simulink model "Kinematics"  (R2022b)
settings: Solver=VariableStepAuto  StartTime=0.0  StopTime=10.0  RelTol=1e-3
libraries: simulink_extras x4
settings Model: Creator=Kumar  LastModifiedBy=Kumar

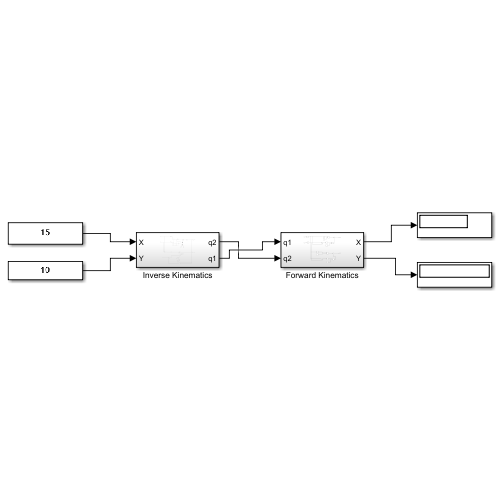
[thumbnail: Simulink's stored preview of the top-level diagram]
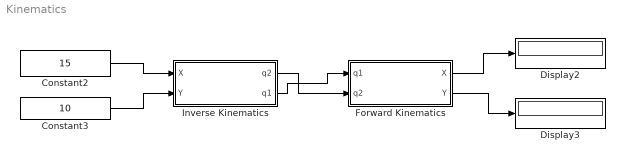
== system Kinematics ==
  Constant2 : Constant  Value=15
  Constant3 : Constant  Value=10
  Display2 : Display
      settings: Format=decimal (Stored Integer)  Decimation=2
  Display3 : Display
      settings: Decimation=2
  Forward Kinematics : Subsystem
  Inverse Kinematics : Subsystem
  wires:
  Constant3/1 -> Inverse Kinematics/2(Y)
  Constant2/1 -> Inverse Kinematics/1(X)
  Forward Kinematics/1(X) -> Display2/1
  Forward Kinematics/2(Y) -> Display3/1
  Inverse Kinematics/1(q2) -> Forward Kinematics/2(q2)
  Inverse Kinematics/2(q1) -> Forward Kinematics/1(q1)

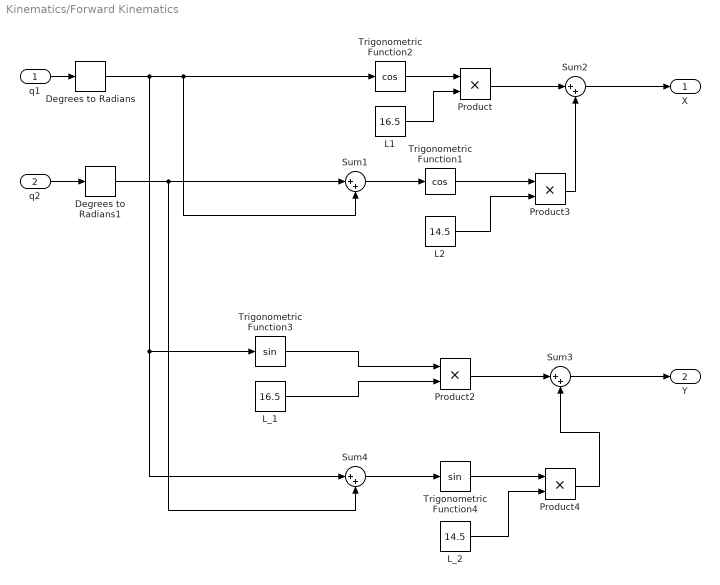
== system Kinematics/Forward Kinematics ==
  q1 : Inport
  q2 : Inport  Port=2
  Degrees to Radians : simulink_extras/Transformations/Degrees to Radians
  Degrees to Radians1 : simulink_extras/Transformations/Degrees to Radians
  L1 : Constant  Value=16.5
  L2 : Constant  Value=14.5
  L_1 : Constant  Value=16.5
  L_2 : Constant  Value=14.5
  Product{,2..4} (4 alike) : Product
  Sum{1..4} (4 alike) : Sum  Inputs=|++
  Trigonometric Function1 : Trigonometry  Operator=cos
  Trigonometric Function2 : Trigonometry  Operator=cos
  Trigonometric Function3 : Trigonometry
  Trigonometric Function4 : Trigonometry
  X : Outport
  Y : Outport  Port=2
  wires:
  Trigonometric Function3/1 -> Product2/1
  q1/1 -> Degrees to Radians/1
  q2/1 -> Degrees to Radians1/1
  Trigonometric Function2/1 -> Product/1
  Trigonometric Function1/1 -> Product3/1
  L1/1 -> Product/2
  Product/1 -> Sum2/1
  L2/1 -> Product3/2
  Product3/1 -> Sum2/2
  Sum1/1 -> Trigonometric Function1/1
  Product2/1 -> Sum3/1
  L_1/1 -> Product2/2
  Sum4/1 -> Trigonometric Function4/1
  Trigonometric Function4/1 -> Product4/1
  Product4/1 -> Sum3/2
  L_2/1 -> Product4/2
  Degrees to Radians/1 -> Trigonometric Function2/1, Sum1/2, Sum4/1, Trigonometric Function3/1
  Degrees to Radians1/1 -> Sum4/2, Sum1/1
  Sum2/1 -> X/1
  Sum3/1 -> Y/1

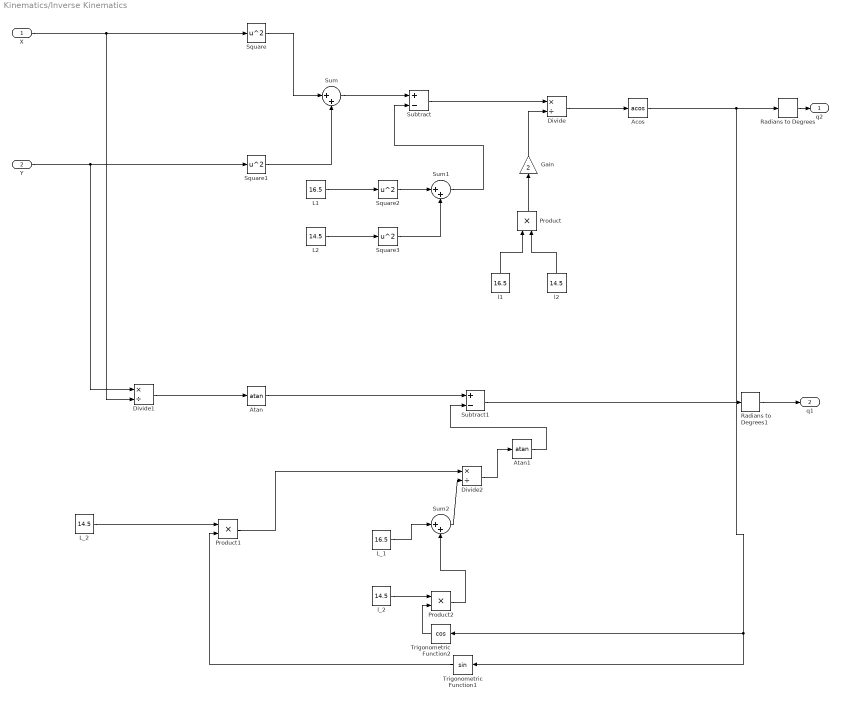
== system Kinematics/Inverse Kinematics ==
  X : Inport
  Y : Inport  Port=2
  Acos : Trigonometry  Operator=acos
  Atan : Trigonometry  Operator=atan
  Atan1 : Trigonometry  Operator=atan
  Divide : Product  Inputs=*/
  Divide1 : Product  Inputs=*/
  Divide2 : Product  Inputs=*/
  Gain : Gain  Gain=2
  L1 : Constant  Value=16.5
  L2 : Constant  Value=14.5
  L_1 : Constant  Value=16.5
  L_2 : Constant  Value=14.5
  Product : Product
  Product1 : Product
  Product2 : Product
  Radians to Degrees : simulink_extras/Transformations/Radians to Degrees
  Radians to Degrees1 : simulink_extras/Transformations/Radians to Degrees
  Square{,1..3} (4 alike) : Math  Operator=square
  Subtract : Sum  Inputs=+-
  Subtract1 : Sum  Inputs=+-
  Sum : Sum  Inputs=|++
  Sum1 : Sum  Inputs=|++
  Sum2 : Sum  Inputs=|++
  Trigonometric Function1 : Trigonometry
  Trigonometric Function2 : Trigonometry  Operator=cos
  l1 : Constant  Value=16.5
  l2 : Constant  Value=14.5
  l_2 : Constant  Value=14.5
  q2 : Outport
  q1 : Outport  Port=2
  wires:
  Square/1 -> Sum/1
  Square1/1 -> Sum/2
  Sum/1 -> Subtract/1
  Sum1/1 -> Subtract/2
  L1/1 -> Square2/1
  L2/1 -> Square3/1
  Square2/1 -> Sum1/1
  Square3/1 -> Sum1/2
  Subtract/1 -> Divide/1
  Divide/1 -> Acos/1
  l1/1 -> Product/1
  l2/1 -> Product/2
  Product/1 -> Gain/1
  Gain/1 -> Divide/2
  Acos/1 -> Radians to Degrees/1, Trigonometric Function2/1, Trigonometric Function1/1
  Divide1/1 -> Atan/1
  Atan/1 -> Subtract1/1
  Subtract1/1 -> Radians to Degrees1/1
  L_2/1 -> Product1/1
  Trigonometric Function1/1 -> Product1/2
  Product1/1 -> Divide2/1
  L_1/1 -> Sum2/1
  Product2/1 -> Sum2/2
  l_2/1 -> Product2/1
  Trigonometric Function2/1 -> Product2/2
  Sum2/1 -> Divide2/2
  X/1 -> Divide1/2, Square/1
  Y/1 -> Divide1/1, Square1/1
  Radians to Degrees/1 -> q2/1
  Radians to Degrees1/1 -> q1/1
  Divide2/1 -> Atan1/1
  Atan1/1 -> Subtract1/2
